simulink model "NN_Test"  (R2019a)
settings: Solver=VariableStepAuto  StartTime=0.0  StopTime=200  RelTol=1e-3
settings Model: Creator=anton  LastModifiedBy=anton

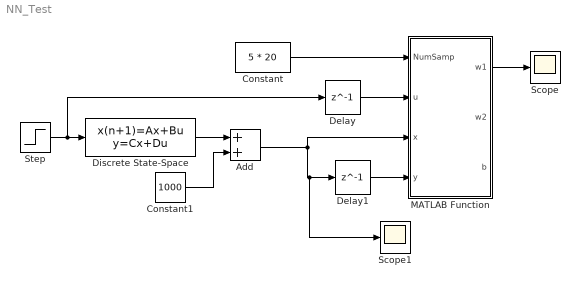
== system NN_Test ==
  Add : Sum
  Constant : Constant  Value=5 * 20
  Constant1 : Constant  Value=1000
  Delay : Delay  DelayLength=1  SampleTime=0.2
  Delay1 : Delay  DelayLength=1  InitialCondition=1000  SampleTime=0.2
  Discrete State-Space : DiscreteStateSpace  A=0.9801  B=3.099e04  D=0  SampleTime=0.2
  MATLAB Function : MATLAB Function  TreatAsAtomicUnit=on
  Scope : Scope
  Scope1 : Scope
  Step : Step  Time=0  After=0.0005  SampleTime=0
  wires:
  Step/1 -> Delay/1, Discrete State-Space/1
  Delay/1 -> MATLAB Function/2(u)
  Delay1/1 -> MATLAB Function/4(y)
  Add/1 -> MATLAB Function/3(x), Scope1/1, Delay1/1
  Constant/1 -> MATLAB Function/1(NumSamp)
  MATLAB Function/1(w1) -> Scope/1
  Discrete State-Space/1 -> Add/1
  Constant1/1 -> Add/2

== matlab function NN_Test/MATLAB Function ==
  settings: updateMethod=DISCRETE  sampleTime=0.2
  data: NumSamp input; w1 output; u input; x input; y input; w2 output; b output
function [w1,w2,b] = fcn(NumSamp,u,x,y)

persistent SampCount
persistent x_buff
persistent y_buff
persistent u_buff

if isempty(SampCount)
    SampCount = 1;
    x_buff = zeros(1,NumSamp);
    y_buff = zeros(1,NumSamp);
    u_buff = zeros(1,NumSamp);  
end

%----------------------------
%AQUIRES DATA FROM SIMULATION
%----------------------------

if(SampCount <= NumSamp)

    x_buff(SampCount) = x;
    u_buff(SampCount) = u;
    y_buff(SampCount) = y;
    
    SampCount = SampCount + 1;    
end

w1 = 0;
w2 = 0;
b = 0;

if(SampCount > NumSamp)
    
    % NEURAL NETWORK TRAINING
    NumInter = 10;
    % NN_Train(x1,x2,y,rate,eps,NumInter)
    [w1,w2,b] = NN_Train(x_buff,u_buff,y_buff,0.001,0.001,NumInter);
    
end
